simulink model "Md57StEnCtrl"  (R2018b)
settings: Solver=FixedStepDiscrete  StartTime=0.0  StopTime=10.0  FixedStep=0.01  RelTol=1e-3
undefined symbols (not defined in the file or in its folder): data, KeSMSuFirstRwStFwdBkwdPosDelta_Val, KeSMSw4SSecRwLtStLgrstUpwdDnwdOpenPos1_Val, PassStBkReclnEn_Clear, PassStBkReclnEn_Set, PassStFldEn_Clear, PassStFldEn_Set, PassStFwdBkwdEn_Clear, PassStFwdBkwdEn_Set, SecRwRtStBkReclnEn_Clear, SecRwRtStBkReclnEn_Set, SecRwRtStFwdBkwdEn_Clear, SecRwRtStFwdBkwdEn_Set, SecRwRtStLgrstInwdOtwdEn_Clear, SecRwRtStLgrstInwdOtwdEn_Set, SecRwRtStLgrstUpwdDnwdEn_Clear, SecRwRtStLgrstUpwdDnwdEn_Set, ThdRwLtStBkReclnEn_Clear, ThdRwLtStBkReclnEn_Set, ThdRwLtStFwdBkwdEn_Clear, ThdRwLtStFwdBkwdEn_Set, ThdRwRtStBkReclnEn_Clear, ThdRwRtStBkReclnEn_Set, ThdRwRtStFwdBkwdEn_Clear, ThdRwRtStFwdBkwdEn_Set, ZeroREn_Clear, ZeroREn_Set
libraries: simulink x1
(part 2 of 2)

== stateflow chart Md57StEnCtrl/Md57StEnCtrl_Cal_sys/Subsystem/Chart ==
  state PosAvlOut=Md57TrgtPosChk [function]
  state [bk,zero,lgrstup,lgrstin,fwd]= Md57trgtPosGet [function]
  (default) -> (junction 205) : {
      | ThdRwLtStBkReclnEn = 0;
      | SecRwLtStBkReclnEn = 0;
      | SecRwLtStFrwdBkwdEn = 0;
      | SecRwLtStLgrstOtwdInwdEn = 0;
      | SecRwLtStLgrstUpwdDnwdEn = 0;
      | ThdRwLtStFwdBkwdEn = 0;
      | ThdRwRtStBkReclnEn = 0;
      | ThdRwRtStFwdBkwdEn = 0;
      | PassStBkReclnEn = 0;
      | PassStFwdBkwdEn = 0;
      | SecRwStZeroEn = 0;
      | PassStFldEn = 0;
      | FwdBkwdFailflg = 0;
      | CshnFldFailflg = 0;
      | }
  (junction 205) -> (junction 207) [order 1] : [FirstTrig]
  (junction 205) -> (junction 211) [order 2]
  (junction 207) -> (junction 209) : {PosAvl=0;}
  (junction 209) -> (junction 211)
  (junction 211) -> (junction 1)
  (junction 1) -> (junction 22) [order 1] : [ThdRwLtStBkReclnStgDone]
  (junction 1) -> (junction 26) [order 2] : {ThdRwLtStBkReclnEn = 1;}
  (junction 22) -> (junction 24)
  (junction 24) -> (junction 26)
  (junction 26) -> (junction 29)
  (junction 29) -> (junction 31) [order 1] : [ThdRwLtStFwdBkwdStgDone]
  (junction 29) -> (junction 35) [order 2] : {
      | ThdRwLtStFwdBkwdEn = 1;
      | }
  (junction 31) -> (junction 33)
  (junction 33) -> (junction 35)
  (junction 35) -> (junction 105)
  (junction 105) -> (junction 109) [order 1] : [ThdRwRtStBkReclnStgDone]
  (junction 105) -> (junction 106) [order 2] : {ThdRwRtStBkReclnEn = 1;}
  (junction 109) -> (junction 110)
  (junction 110) -> (junction 106)
  (junction 106) -> (junction 108)
  (junction 108) -> (junction 117) [order 1] : [ThdRwRtStFwdBkwdStgDone]
  (junction 108) -> (junction 107) [order 2] : {
      | ThdRwRtStFwdBkwdEn = 1;
      | }
  (junction 117) -> (junction 114)
  (junction 114) -> (junction 107)
  (junction 107) -> (junction 124)
  (junction 124) -> (junction 126) [order 1] : [NotMovPassStFlg]
  (junction 124) -> (junction 252) [order 2]
  (junction 126) -> (junction 129)
  (junction 252) -> (junction 253) [order 1] : [PassStFwdBkwdStgDone ]
  (junction 253) -> (junction 254) [order 1] : [(PassStFwdBkwdPos<(PassStFwdBkwdTrgtPos1-KeSMSuFirstRwStFwdBkwdPosDelta))&&!PassStBkReclnStgDone]
  (junction 252) -> (junction 255) [order 2] : {PassStFwdBkwdEn = 1;}
  (junction 253) -> (junction 258) [order 2]
  (junction 254) -> (junction 257) : {FwdBkwdFailflg =1;}
  (junction 258) -> (junction 255)
  (junction 257) -> (junction 258)
  (junction 255) -> (junction 256)
  (junction 256) -> (junction 261) [order 1] : [PassStFwdBkwdPos>=(PassStFwdBkwdTrgtPos1-KeSMSuFirstRwStFwdBkwdPosDelta)]
  (junction 261) -> (junction 263) [order 1] : [PassStFldStgDone ]
  (junction 263) -> (junction 264) [order 1] : [PassStFldUpwdDnwdPos >PassStCshnFldTrgtPos1]
  (junction 256) -> (junction 238) [order 2]
  (junction 261) -> (junction 265) [order 2] : {
      | PassStFldEn = 1;
      | }
  (junction 263) -> (junction 262) [order 2]
  (junction 264) -> (junction 224) : {
      | CshnFldFailflg = 1;
      | }
  (junction 262) -> (junction 265)
  (junction 265) -> (junction 259)
  (junction 259) -> (junction 260) [order 1] : [(PassStFldUpwdDnwdPos <=PassStCshnFldTrgtPos1)&&!PassStBkReclnStgDone]
  (junction 259) -> (junction 237) [order 2]
  (junction 260) -> (junction 239) : {PassStBkReclnEn = 1;}
  (junction 237) -> (junction 238)
  (junction 239) -> (junction 237)
  (junction 224) -> (junction 239)
  (junction 129) -> (junction 224)
  (junction 238) -> (junction 153)
  (junction 153) -> (junction 157) [order 1] : [Stg1Done]
  (junction 157) -> (junction 216) [order 1] : [!PosAvl]
  (junction 153) -> (junction 166) [order 2]
  (junction 157) -> (junction 220) [order 2]
  (junction 216) -> (junction 218) : {PosAvl = Md57TrgtPosChk ();}
  (junction 218) -> (junction 220)
  (junction 220) -> (junction 159)
  (junction 159) -> (junction 38) [order 1] : [PosAvl]
  (junction 159) -> (junction 169) [order 2]
  (junction 38) -> (junction 196) : {[bktrgt,zerotrgt,lgrstuptrgt,lgrstintrgt,fwdtrgt]=Md57trgtPosGet();}
  (junction 196) -> (junction 40) [order 1] : [IfVeSMSuSecRwLtStBkReclnUpwdDnwdPos>bktrgt&&!SecRwLtStBkReclnStgDone]
  (junction 196) -> (junction 44) [order 2]
  (junction 40) -> (junction 42) : {SecRwLtStBkReclnEn = 1;}
  (junction 42) -> (junction 44)
  (junction 44) -> (junction 47)
  (junction 47) -> (junction 49) [order 1] : [IfVeSMSuSecRwLtStLgrstOtwdInwdPos >lgrstintrgt &&!SecRwLtStLgrstOtwdInwdStgDone]
  (junction 47) -> (junction 53) [order 2]
  (junction 49) -> (junction 51) : {SecRwLtStLgrstOtwdInwdEn = 1;}
  (junction 51) -> (junction 53)
  (junction 53) -> (junction 56)
  (junction 56) -> (junction 58) [order 1] : [IfVeSMSuSecRwLtStLgrstUpwdDnwdPos >lgrstuptrgt && !SecRwLtStLgrstUpwdDnwdStgDone]
  (junction 56) -> (junction 62) [order 2]
  (junction 58) -> (junction 60) : {SecRwLtStLgrstUpwdDnwdEn = 1;}
  (junction 60) -> (junction 62)
  (junction 62) -> (junction 172)
  (junction 172) -> (junction 174) [order 1] : [IfVeSMSuSecRwRtStZeroPos >zerotrgt && !ZeroRStgDone]
  (junction 172) -> (junction 178) [order 2]
  (junction 174) -> (junction 176) : {SecRwStZeroEn = 1; }
  (junction 176) -> (junction 178)
  (junction 178) -> (junction 65)
  (junction 65) -> (junction 67) [order 1] : [
      | (IfVeSMSuSecRwLtStBkReclnUpwdDnwdPos<=bktrgt||SecRwLtStBkReclnStgDone)&&...
      | (IfVeSMSuSecRwLtStLgrstOtwdInwdPos <=lgrstintrgt ||SecRwLtStLgrstOtwdInwdStgDone) &&...
      | (IfVeSMSuSecRwLtStLgrstUpwdDnwdPos <=lgrstuptrgt ||SecRwLtStLgrstUpwdDnwdStgDone)&&...
      | (IfVeSMSuSecRwRtStZeroPos <=zerotrgt || ZeroRStgDone)
      | ]
  (junction 67) -> (junction 69) [order 1] : [SecRwLtStFrwdBkwdStgDone]
  (junction 69) -> (junction 76) [order 1] : [SecRwLtStBkReclnStgDone]
  (junction 65) -> (junction 87) [order 2]
  (junction 67) -> (junction 73) [order 2] : {SecRwLtStFrwdBkwdEn =1;}
  (junction 69) -> (junction 71) [order 2] : {SecRwLtStBkReclnEn = 1;}
  (junction 76) -> (junction 78)
  (junction 78) -> (junction 71)
  (junction 71) -> (junction 181)
  (junction 181) -> (junction 183) [order 1] : [ZeroRStgDone]
  (junction 181) -> (junction 187) [order 2] : {SecRwStZeroEn = 1; }
  (junction 183) -> (junction 185)
  (junction 185) -> (junction 187)
  (junction 187) -> (junction 81) : {LgrstOpn;}
  (junction 169) -> (junction 166)
  (junction 87) -> (junction 169)
  (junction 73) -> (junction 87)
  (junction 81) -> (junction 73)
  data: PosAvlOut function_output; bk function_output; zero function_output; lgrstup function_output; lgrstin function_output; fwd function_output; IfVeSMSuSecRwLtStBkReclnUpwdDnwdPos input; IfVeSMSuSecRwLtStLgrstOtwdInwdPos input; IfVeSMSuSecRwLtStLgrstUpwdDnwdPos input; SecRwLtStBkReclnStgDone input; SecRwLtStFrwdBkwdStgDone input; SecRwLtStLgrstOtwdInwdStgDone input; SecRwLtStLgrstUpwdDnwdStgDone input; ThdRwLtStBkReclnStgDone input; ThdRwLtStFwdBkwdStgDone input; VIPLR2LBkReclnUpwdDnwdTrgtPos input; VIPLR2LFwdBkwdTrgtPos input; VIPLR2LLgrstInwdOtwdTrgtPos input; VIPLR2LLgrstUpwdDnwdTrgtPos input; SecRwLtStBkReclnEn output boolean; SecRwLtStFrwdBkwdEn output boolean; SecRwLtStLgrstOtwdInwdEn output boolean; ThdRwLtStBkReclnEn output boolean; ThdRwLtStFwdBkwdEn output boolean; SecRwLtStLgrstUpwdDnwdEn output boolean; ThdRwRtStBkReclnEn output boolean; ThdRwRtStFwdBkwdEn output boolean; PassStBkReclnEn output boolean; PassStFwdBkwdEn output boolean; ThdRwRtStBkReclnStgDone input; ThdRwRtStFwdBkwdStgDone input; PassStBkReclnStgDone input; PassStFwdBkwdStgDone input; NotMovPassStFlg input boolean; NotMovPassStBkReclnFlg input boolean; IfVeSMSuSecRwRtStZeroPos input; VIPRMdR2RZeroTrgtPos input; ZeroRStgDone input boolean; Stg1Done input boolean; SecRwStZeroEn output boolean; PosAvl output boolean; bktrgt local uint16; zerotrgt local uint16; lgrstuptrgt local uint16; lgrstintrgt local uint16; fwdtrgt local uint16; FirstTrig input boolean; PassStFldEn output boolean; PassStFwdBkwdTrgtPos1 input; KeSMSuFirstRwStFwdBkwdPosDelta input; PassStCshnFldTrgtPos1 input; FwdBkwdFailflg output boolean; CshnFldFailflg output boolean; PassStFldUpwdDnwdPos input; PassStFwdBkwdPos input; PassStFldStgDone input
  events: LgrstOpn output FUNCTION_CALL_EVENT
